simulink model "Parametres_ModeleCausal_2017a"  (R2017a)
settings: Solver=VariableStepAuto  StartTime=0.0  StopTime=3  FixedStep=0.01  RelTol=1e-5
values from neighbouring files (symbols this model uses):
  f = 0.00333529843887    [Workspace_Simulink_final.mat]    (also in Workspace_Simulink_initial.mat = 0.006)
  J = 0.00108207552857    [Workspace_Simulink_final.mat]    (also in Workspace_Simulink_initial.mat = 0.002)
  Ke = 0.1    [Workspace_Simulink_final.mat]    (also in Workspace_Simulink_initial.mat)
  L = 0.162408641357    [Workspace_Simulink_final.mat]    (also in Workspace_Simulink_initial.mat = 0.1)
  R = 2.990841745    [Workspace_Simulink_final.mat]    (also in Workspace_Simulink_initial.mat = 2)
settings Model: Creator=carmen  LastModifiedBy=carmen
settings DataIOCC: ExternalInput=[time_IN,Signal_IN]  LoadExternalInput=on  SaveFormat=Array  SaveOutput=off  SaveTime=off  TimeSaveName=time1  OutputTimes=SDO_OutputTimes
settings SFSimCC: SimUseLocalCustomCode=on
settings RTWCC: RTWUseLocalCustomCode=on

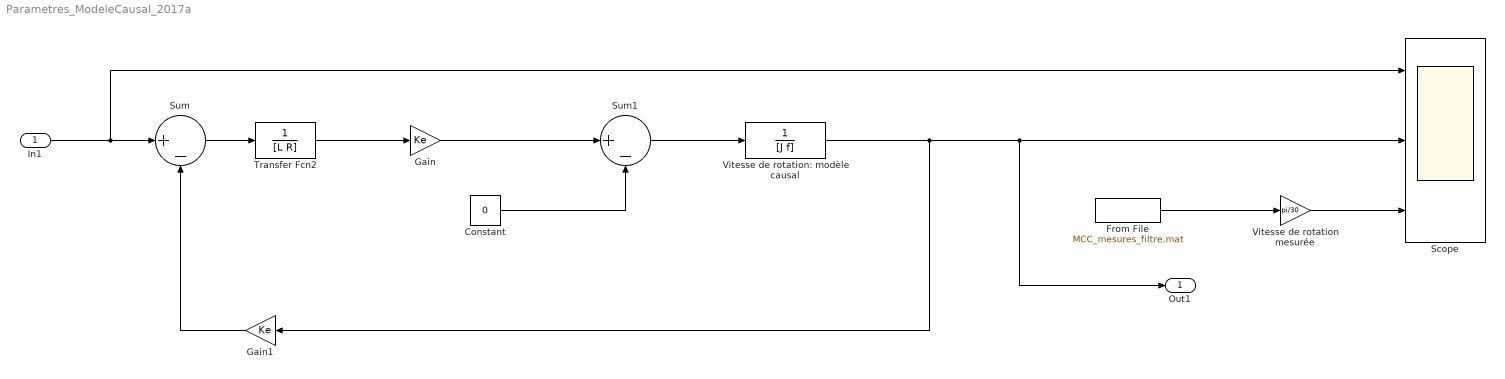
== system Parametres_ModeleCausal_2017a ==
  In1 : Inport
  Constant : Constant  Value=0
  From File : FromFile  FileName=MCC_mesures_filtre.mat  OutDataTypeStr=double  SampleTime=0.01
  Gain : Gain  Gain=Ke
  Gain1 : Gain  Gain=Ke
  Scope : Scope  NumInputPorts=3
  Sum : Sum  Inputs=|+-
  Sum1 : Sum  Inputs=|+-
  Transfer Fcn2 : TransferFcn  Denominator=[L R]
  Vitesse de rotation mesurée : Gain  Gain=pi/30
  Vitesse de rotation: modèle causal : TransferFcn  Denominator=[J f]
  Out1 : Outport
  wires:
  Sum/1 -> Transfer Fcn2/1
  Transfer Fcn2/1 -> Gain/1
  Vitesse de rotation: modèle causal/1 -> Scope/2, Out1/1, Gain1/1
  Gain1/1 -> Sum/2
  Constant/1 -> Sum1/2
  Gain/1 -> Sum1/1
  Sum1/1 -> Vitesse de rotation: modèle causal/1
  From File/1 -> Vitesse de rotation mesurée/1
  In1/1 -> Scope/1, Sum/1
  Vitesse de rotation mesurée/1 -> Scope/3
